simulink model "vector_loop_alt"  (R2022a)
settings: Solver=ode45  StartTime=0.0  StopTime=1.5  RelTol=1e-9
undefined symbols (not defined in the file or in its folder): BikeKin
settings Model: PacingRate=0.001600  Creator=jason  LastModifiedBy=Jason

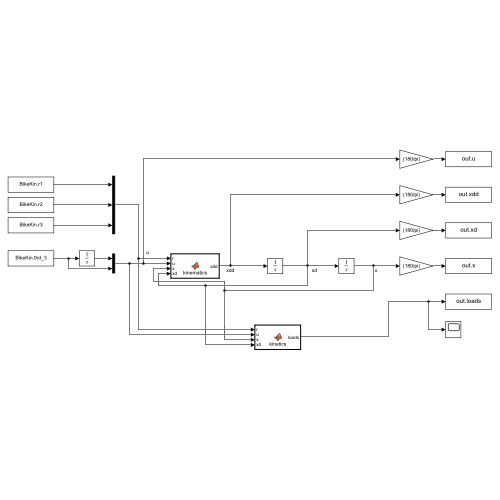
[thumbnail: Simulink's stored preview of the top-level diagram]
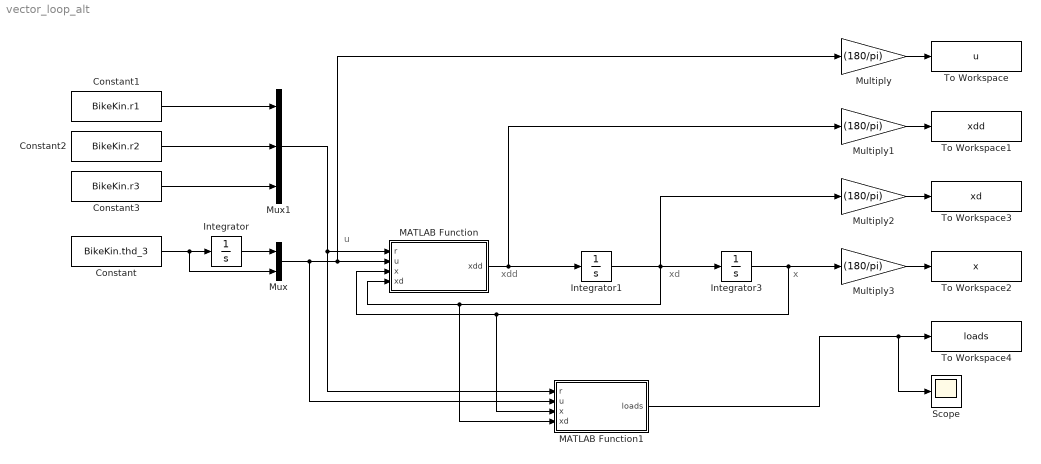
== system vector_loop_alt ==
  note: u
  note: xdd
  note: xd
  note: x
  Constant : Constant  Value=BikeKin.thd_3
  Constant1 : Constant  Value=BikeKin.r1
  Constant2 : Constant  Value=BikeKin.r2
  Constant3 : Constant  Value=BikeKin.r3
  Integrator : Integrator  InitialCondition=BikeKin.th3
  Integrator1 : Integrator  InitialCondition=BikeKin.statevectord
  Integrator3 : Integrator  InitialCondition=BikeKin.statevector
  MATLAB Function : MATLAB Function  TreatAsAtomicUnit=on
  MATLAB Function1 : MATLAB Function  TreatAsAtomicUnit=on
  Multiply{,1..3} (4 alike) : Gain  Gain=(180/pi)
  Mux : Mux  Inputs=2
  Mux1 : Mux  Inputs=3
  Scope : Scope
  To Workspace : ToWorkspace  VariableName=u  SampleTime=-1
  To Workspace1 : ToWorkspace  VariableName=xdd  SampleTime=-1
  To Workspace2 : ToWorkspace  VariableName=x  SampleTime=-1
  To Workspace3 : ToWorkspace  VariableName=xd  SampleTime=-1
  To Workspace4 : ToWorkspace  VariableName=loads  SampleTime=-1
  wires:
  Integrator/1 -> Mux/1
  Mux/1 -> MATLAB Function1/2(u), MATLAB Function/2(u), Multiply/1
  Integrator1/1 -> MATLAB Function1/4(xd), MATLAB Function/4(xd), Multiply2/1, Integrator3/1
  Integrator3/1 -> MATLAB Function1/3(x), MATLAB Function/3(x), Multiply3/1
  MATLAB Function/1(xdd) -> Multiply1/1, Integrator1/1
  Constant/1 -> Mux/2, Integrator/1
  Multiply/1 -> To Workspace/1
  Multiply1/1 -> To Workspace1/1
  Multiply2/1 -> To Workspace3/1
  Multiply3/1 -> To Workspace2/1
  Mux1/1 -> MATLAB Function1/1(r), MATLAB Function/1(r)
  Constant3/1 -> Mux1/3
  Constant2/1 -> Mux1/2
  Constant1/1 -> Mux1/1
  MATLAB Function1/1(loads) -> Scope/1, To Workspace4/1

== matlab function vector_loop_alt/MATLAB Function1 ==
  data: r input; u input; loads output; x input; xd input
function loads = kinetics(r,u,x,xd)
% K_x, K_y, M_k = 0;

% System Constants
m_body = 67.132;        % kg
m_s = 0.097 * m_body;   % kg
a_g = 9.81;             % m/s^2

% Lengths
r1 = r(1);              % m
r2 = r(2);              % m
r3 = r(3);              % m
g2 = 0.43*r2;           % m

% Angles
% All angles imported from Matlab live script and have been preconverted to
% radians, rad/s
% They are converted back to degrees in Simulink
th3 = u(1);
thd_3 = u(2);

th1 = x(1);
th2 = x(2);
thd_1 = xd(1);
thd_2 = xd(2);

%  Vector Components
s1 = sin(th1);
s2 = sin(th2);
s3 = sin(th3);

c1 = cos(th1);
c2 = cos(th2);
c3 = cos(th3);

% Matrix algebra
A1 = [-r1*s1 -r2*s2
       r1*c1 r2*c2];

b1 = [r1*c1*(thd_1^2)+r2*c2*(thd_2^2)+r3*c3*(thd_3^2)
      r1*s1*(thd_1^2)+r2*s2*(thd_2^2)+r3*s3*(thd_3^2)];

xdd = A1\b1;
thdd_2 = xdd(2);

% Moments of Inertia
I_G2 = (m_s)*(r2^2)*(0.323^2);  % kg*m^2

% Pedal forces
P = [(-90 * sin(th3 + 1.5708) - 30)
     (160 * sin(th3 - 0.5236) + 160)];

% Acceleration Analysis
r_PC = [r3*c3 r3*s3 0];
r_GP = [(r2-g2)*c2 (r2-g2)*s2 0];
r_KP = [r2*c2 r2*s2 0]; 

omega_PC = [0 0 thd_3];
alpha_PC = [0 0 0];

omega_GP = [0 0 thd_2];
alpha_GP = [0 0 thdd_2];

% Relative Acceleration Analysis
a_C = [0 0 0];
a_P = relA(a_C, omega_PC, alpha_PC, r_PC);
a_G = relA(a_P, omega_GP, alpha_GP, r_GP);

A2 = [-1 0 0 1 0
      0 -1 0 0 1
      (g2*s2) (-g2*c2) -1 ((r2-g2)*s2) (-(r2-g2)*(c2))
      0 0 0 1 0
      0 0 0 0 1];

b2 = [m_s*a_G(1)
      m_s*(a_G(2) +  a_g)
      -I_G2*thdd_2
      P(1)
      P(2)];

loads = A2\b2;

% loads = [K_x
%          K_y
%          M_k
%          P(1)
%          P(2)];

end

== matlab function vector_loop_alt/MATLAB Function ==
  data: r input; u input; xdd output; x input; xd input
function xdd = kinematics(r, u, x, xd)
% function xdd = fcn(r, u, x, xd)

% K_x, K_y, M_k = 0;

% System Constants
m_body = 67.132;        % kg
m_s = 0.097 * m_body;   % kg
a_g = 9.81;               % m/s^2

% Lengths
r1 = r(1);              % m
r2 = r(2);              % m
r3 = r(3);              % m
g2 = 0.43*r2;           % m

% Angles
% All angles imported from Matlab live script and have been preconverted to
% radians, rad/s
% They are converted back to degrees in Simulink
th3 = u(1);
thd_3 = u(2);

th1 = x(1);
th2 = x(2);
thd_1 = xd(1);
thd_2 = xd(2);

%  Vector Components
s1 = sin(th1);
s2 = sin(th2);
s3 = sin(th3);

c1 = cos(th1);
c2 = cos(th2);
c3 = cos(th3);

% Matrix algebra
A2 = [-r1*s1 -r2*s2
       r1*c1 r2*c2];

b2 = [r1*c1*(thd_1^2)+r2*c2*(thd_2^2)+r3*c3*(thd_3^2)
      r1*s1*(thd_1^2)+r2*s2*(thd_2^2)+r3*s3*(thd_3^2)];

xdd = A2\b2;
thdd_2 = xdd(2);

% Moments of Inertia
I_G2 = (m_s)*(r2^2)*(0.323^2);  % kg*m^2

% Moment of inertia about K (Parallel Axis Thm)
I_K = I_G2 + m_s*g2^2;               % kg*m^2

P = [(-90 * sin(th3 + 1.5708) - 30)
     (160 * sin(th3 - 0.5236) + 160)];

% Moments
M_1 = abs(P(1)*r2*c2);
M_2 = abs(m_s*a_g*g2*s2);
M_3 = abs(P(2)*r2*s2);
M_4 = abs(I_K)*thdd_2;

K_x = P(1) + m_s*r2*c2*thd_2^2 + m_s*r3*c3*thd_3^2 + m_s*r2*s2*thdd_2;
K_y = P(2) - m_s*a_g + m_s*r2*s2*thd_2^2 + m_s*r3*s3*thd_3^2 -m_s*r2*c2*thdd_2;
M_k = M_1 + M_2 - M_3 - M_4;

loads = [K_x
         K_y
         M_k
         P(1)
         P(2)];

end
